simulink model "Pemodelan_Matematis_Boost_Converter"  (R2019a)
settings: Solver=VariableStepAuto  StartTime=0.0  StopTime=0.1  RelTol=1e-3
undefined symbols (not defined in the file): C, L, R
settings Model: Creator=Farizbot  LastModifiedBy=Farizbot

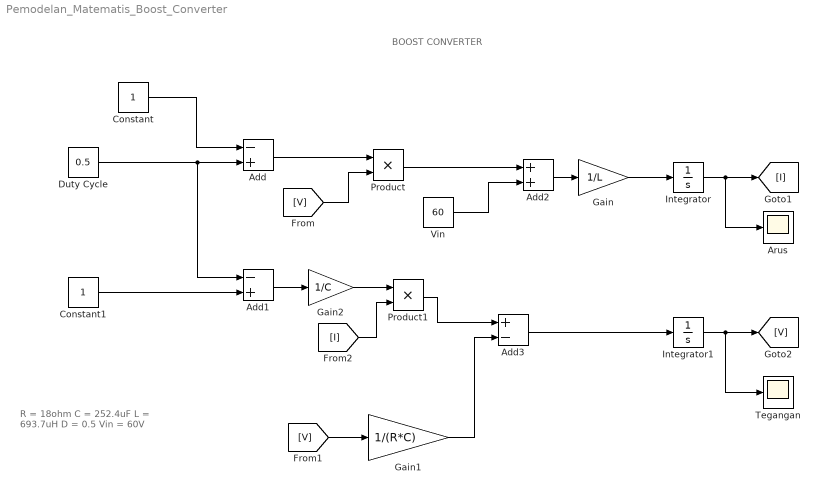
== system Pemodelan_Matematis_Boost_Converter ==
  note: R = 18ohm
      | C = 252.4uF
      | L = 693.7uH
      | D = 0.5
      | Vin = 60V
  note: BOOST CONVERTER
  Add : Sum  Inputs=-+
  Add1 : Sum  Inputs=-+
  Add2 : Sum
  Add3 : Sum  Inputs=+-
  Arus : Scope
  Constant : Constant
  Constant1 : Constant
  Duty Cycle : Constant  Value=0.5
  Gain : Gain  Gain=1/L
  Gain1 : Gain  Gain=1/(R*C)
  Gain2 : Gain  Gain=1/C
  Integrator : Integrator
  Integrator1 : Integrator
  Product : Product
  Product1 : Product
  Tegangan : Scope
  Vin : Constant  Value=60
  wires:
  Duty Cycle/1 -> Add1/1, Add/2
  Constant/1 -> Add/1
  Constant1/1 -> Add1/2
  Add2/1 -> Gain/1
  Gain/1 -> Integrator/1
  Integrator/1 -> Arus/1, [I]
  Vin/1 -> Add2/2
  Add/1 -> Product/1
  Product/1 -> Add2/1
  [V] -> Product/2
  [V] -> Gain1/1
  Gain1/1 -> Add3/2
  Add1/1 -> Gain2/1
  Gain2/1 -> Product1/1
  [I] -> Product1/2
  Product1/1 -> Add3/1
  Add3/1 -> Integrator1/1
  Integrator1/1 -> Tegangan/1, [V]
